simulink model "task_9"  (R2022b)
settings: Solver=VariableStepAuto  StartTime=0.0  StopTime=10.0  RelTol=1e-3
values from neighbouring files (symbols this model uses):
  Kp = place(A,B,polc)    [kod.m]
undefined symbols (not defined in the file or in its folder): A, B, C
settings Model: Creator=mrxmi  LastModifiedBy=mrxmi

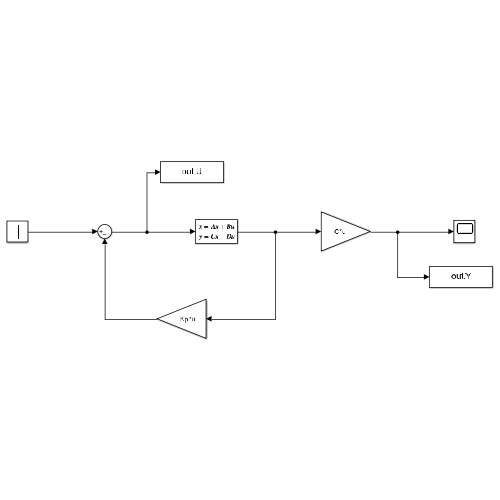
[thumbnail: Simulink's stored preview of the top-level diagram]
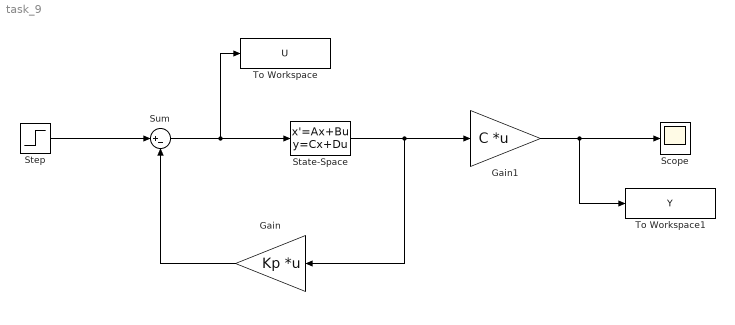
== system task_9 ==
  Gain : Gain  Gain=Kp  Multiplication=Matrix(K*u)
  Gain1 : Gain  Gain=C  Multiplication=Matrix(K*u)
  Scope : Scope
  State-Space : StateSpace  A=A  B=B  C=eye(5)  D=zeros(5,1)  InitialCondition=0
  Step : Step  SampleTime=0
  Sum : Sum  Inputs=|+-
  To Workspace : ToWorkspace  VariableName=U  SampleTime=-1
  To Workspace1 : ToWorkspace  VariableName=Y  SampleTime=-1
  wires:
  State-Space/1 -> Gain/1, Gain1/1
  Sum/1 -> To Workspace/1, State-Space/1
  Step/1 -> Sum/1
  Gain1/1 -> To Workspace1/1, Scope/1
  Gain/1 -> Sum/2
